simulink model "Manu6DOF_MICO_NE_v6articulation2019b"  (R2019b)
settings: Solver=ode5  StartTime=0.0  StopTime=10.0  FixedStep=0.001  RelTol=1e-3
undefined symbols (not defined in the file): f, Sub02MIHM
libraries: instrumentlib x27, dspnetwork x24, simulink x7, dspmtrx3 x3, dspsrcs4 x1
(part 3 of 3)

== matlab function Manu6DOF_MICO_NE_v6articulation2019b/Nmm to Nm ==
  data: qm input; T output
function T = fcn(qm)
%Newton milimeter to Newton meter

t1 = qm(1);
t2 = qm(2);
t3 = qm(3);
t4 = qm(4);
t5 = qm(5);
t6 = qm(6);


T = [t1*0.001;t2*0.001;t3*0.001;t4*0.001;t5*0.001;t6*0.001];

%%

== matlab function Manu6DOF_MICO_NE_v6articulation2019b/D ==
  data: qm input; M output
function M = fcn(qm)

q1 = qm(1);
q2 = qm(2);
q3 = qm(3);
q4 = qm(4);
q5 = qm(5);
q6 = qm(6);

%%%%%%%
%function M = M(q1,q2,q3,q4,q5,q6)
%D_Q

%    This function was generated by the Symbolic Math Toolbox version 8.4.
%    09-Jul-2020 20:13:24

M = reshape([conj(q1).*(-1.571066306042153e+4)-conj(q2).*4.088711718154727e+4+conj(q3).*6.059193811420593e+5+conj(q4).*2.254880071272725e+5-conj(q5).*2.343560231418765e+5+conj(q6).*2.101846903564805e+5+conj(q1).*conj(q2).*2.99983383266e+3+conj(q1).*conj(q3).*1.317626777332713e-13+conj(q1).*conj(q4).*5.296107547592644e-14+conj(q2).*conj(q3).*1.317626777332713e-13-conj(q1).*conj(q5).*4.873849331246636e-14+conj(q2).*conj(q4).*5.296107547592644e-14+conj(q1).*conj(q6).*1.335477334470189e-13-conj(q2).*conj(q5).*4.873849331246636e-14+conj(q3).*conj(q4).*8.6492e+2+conj(q2).*conj(q6).*1.335477334470189e-13-conj(q3).*conj(q5).*7.9596e+2+conj(q3).*conj(q6).*7.27e+2+conj(q4).*conj(q5).*7.9596e+2-conj(q4).*conj(q6).*7.27e+2-conj(q5).*conj(q6).*1.454e+3+conj(q1).^2.*1.68190091725e+3+conj(q2).^2.*1.49991691633e+3+conj(q3).^2.*1.07592391394e+3+conj(q4).^2.*8.6492e+2+conj(q5).^2.*7.9596e+2+conj(q6).^2.*7.27e+2+sqrt(3.0).*1.67928161329898e+7+sqrt(3.0).*conj(q1).*1.015019680000001e+4+sqrt(3.0).*conj(q2).*1.015019680000001e+4+sqrt(3.0).*conj(q3).*6.09614312e+4+sqrt(3.0).*conj(q4).*6.036768560000001e+4+sqrt(3.0).*conj(q5).*1.309327791027026e-11-sqrt(3.0).*conj(q6).*3.645574198348217e-11+sqrt(3.0).*conj(q4).^2.*2.902843497617834e-31-sqrt(3.0).*conj(q5).^2.*2.671400025856601e-31-sqrt(3.0).*conj(q6).^2.*7.319869662286102e-31-sqrt(3.0).*conj(q1).*conj(q4).*8.6492e+2-sqrt(3.0).*conj(q1).*conj(q5).*7.9596e+2-sqrt(3.0).*conj(q2).*conj(q4).*8.6492e+2+sqrt(3.0).*conj(q1).*conj(q6).*7.27e+2-sqrt(3.0).*conj(q2).*conj(q5).*7.9596e+2+sqrt(3.0).*conj(q3).*conj(q4).*5.805686995235668e-31+sqrt(3.0).*conj(q2).*conj(q6).*7.27e+2+sqrt(3.0).*conj(q3).*conj(q5).*5.342800051713201e-31-sqrt(3.0).*conj(q3).*conj(q6).*8.903182229801258e-14-sqrt(3.0).*conj(q4).*conj(q6).*8.903182229801258e-14+sqrt(3.0).*conj(q5).*conj(q6).*9.75982621638147e-31+1.141163110828982e+8,conj(q1).*(-2.044355859077363e+4)-conj(q2).*4.088711718154727e+4+conj(q3).*3.095751114833673e+5+conj(q4).*1.063745259636362e+5-conj(q5).*1.247394499709383e+5+conj(q6).*1.100650251782402e+5+conj(q1).*conj(q2).*1.49991691633e+3+conj(q1).*conj(q3).*6.588133886663567e-14+conj(q1).*conj(q4).*2.648053773796322e-14+conj(q2).*conj(q3).*1.317626777332713e-13-conj(q1).*conj(q5).*2.436924665623318e-14+conj(q2).*conj(q4).*5.296107547592644e-14+conj(q1).*conj(q6).*6.677386672350943e-14-conj(q2).*conj(q5).*4.873849331246636e-14+conj(q3).*conj(q4).*8.6492e+2+conj(q2).*conj(q6).*1.335477334470189e-13-conj(q3).*conj(q5).*7.9596e+2+conj(q3).*conj(q6).*7.27e+2+conj(q4).*conj(q5).*7.9596e+2-conj(q4).*conj(q6).*7.27e+2-conj(q5).*conj(q6).*1.454e+3+conj(q2).^2.*1.49991691633e+3+conj(q3).^2.*1.07592391394e+3+conj(q4).^2.*8.6492e+2+conj(q5).^2.*7.9596e+2+conj(q6).^2.*7.27e+2+sqrt(3.0).*8.397440506400625e+6+sqrt(3.0).*conj(q1).*5.075098400000006e+3+sqrt(3.0).*conj(q2).*1.015019680000001e+4+sqrt(3.0).*conj(q3).*6.09614312e+4+sqrt(3.0).*conj(q4).*6.036768560000001e+4+sqrt(3.0).*conj(q5).*6.381198636905707e-12-sqrt(3.0).*conj(q6).*1.806405785964667e-11+sqrt(3.0).*conj(q4).^2.*2.902843497617834e-31-sqrt(3.0).*conj(q5).^2.*2.671400025856601e-31-sqrt(3.0).*conj(q6).^2.*7.319869662286102e-31-sqrt(3.0).*conj(q1).*conj(q4).*4.3246e+2-sqrt(3.0).*conj(q1).*conj(q5).*3.9798e+2-sqrt(3.0).*conj(q2).*conj(q4).*8.6492e+2+sqrt(3.0).*conj(q1).*conj(q6).*3.635e+2-sqrt(3.0).*conj(q2).*conj(q5).*7.9596e+2+sqrt(3.0).*conj(q3).*conj(q4).*5.805686995235668e-31+sqrt(3.0).*conj(q2).*conj(q6).*7.27e+2+sqrt(3.0).*conj(q3).*conj(q5).*5.342800051713201e-31-sqrt(3.0).*conj(q3).*conj(q6).*8.903182229801258e-14-sqrt(3.0).*conj(q4).*conj(q6).*8.903182229801258e-14+sqrt(3.0).*conj(q5).*conj(q6).*9.75982621638147e-31+2.944694702731556e+7,conj(q1).*(-2.990189516772894e+4)-conj(q2).*2.990189516772894e+4+conj(q3).*3.095751114833673e+5+conj(q4).*1.063745259636362e+5-conj(q5).*1.247394499709383e+5+conj(q6).*1.100650251782402e+5+conj(q1).*conj(q3).*6.588133886663567e-14+conj(q1).*conj(q4).*2.648053773796322e-14+conj(q2).*conj(q3).*6.588133886663567e-14-conj(q1).*conj(q5).*2.436924665623318e-14+conj(q2).*conj(q4).*2.648053773796322e-14+conj(q1).*conj(q6).*6.677386672350943e-14-conj(q2).*conj(q5).*2.436924665623318e-14+conj(q3).*conj(q4).*8.6492e+2+conj(q2).*conj(q6).*6.677386672350943e-14-conj(q3).*conj(q5).*7.9596e+2+conj(q3).*conj(q6).*7.27e+2+conj(q4).*conj(q5).*7.9596e+2-conj(q4).*conj(q6).*7.27e+2-conj(q5).*conj(q6).*1.454e+3+conj(q3).^2.*1.07592391394e+3+conj(q4).^2.*8.6492e+2+conj(q5).^2.*7.9596e+2+conj(q6).^2.*7.27e+2+sqrt(3.0).*8.395359070654554e+6+sqrt(3.0).*conj(q1).*5.075098400000006e+3+sqrt(3.0).*conj(q2).*5.075098400000006e+3+sqrt(3.0).*conj(q3).*6.09614312e+4+sqrt(3.0).*conj(q4).*6.036768560000001e+4+sqrt(3.0).*conj(q5).*6.381198636905707e-12-sqrt(3.0).*conj(q6).*1.806405785964667e-11+sqrt(3.0).*conj(q4).^2.*2.902843497617834e-31-sqrt(3.0).*conj(q5).^2.*2.671400025856601e-31-sqrt(3.0).*conj(q6).^2.*7.319869662286102e-31-sqrt(3.0).*conj(q1).*conj(q4).*4.3246e+2-sqrt(3.0).*conj(q1).*conj(q5).*3.9798e+2-sqrt(3.0).*conj(q2).*conj(q4).*4.3246e+2+sqrt(3.0).*conj(q1).*conj(q6).*3.635e+2-sqrt(3.0).*conj(q2).*conj(q5).*3.9798e+2+sqrt(3.0).*conj(q3).*conj(q4).*5.805686995235668e-31+sqrt(3.0).*conj(q2).*conj(q6).*3.635e+2+sqrt(3.0).*conj(q3).*conj(q5).*5.342800051713201e-31-sqrt(3.0).*conj(q3).*conj(q6).*8.903182229801258e-14-sqrt(3.0).*conj(q4).*conj(q6).*8.903182229801258e-14+sqrt(3.0).*conj(q5).*conj(q6).*9.75982621638147e-31+7.050641110794516e+6,conj(q1).*(-2.988697e+4)-conj(q2).*2.988697e+4+conj(q3).*2.486340000000004e+3+conj(q4).*1.063745259636362e+5-conj(q5).*1.247394499709383e+5+conj(q6).*1.100650251782402e+5+conj(q1).*conj(q4).*2.648053773796322e-14-conj(q1).*conj(q5).*2.436924665623318e-14+conj(q2).*conj(q4).*2.648053773796322e-14+conj(q1).*conj(q6).*6.677386672350943e-14-conj(q2).*conj(q5).*2.436924665623318e-14+conj(q3).*conj(q4).*4.3246e+2+conj(q2).*conj(q6).*6.677386672350943e-14-conj(q3).*conj(q5).*3.9798e+2+conj(q3).*conj(q6).*3.635e+2+conj(q4).*conj(q5).*7.9596e+2-conj(q4).*conj(q6).*7.27e+2-conj(q5).*conj(q6).*1.454e+3+conj(q4).^2.*8.6492e+2+conj(q5).^2.*7.9596e+2+conj(q6).^2.*7.27e+2+sqrt(3.0).*8.395359070654554e+6+sqrt(3.0).*conj(q1).*5.075098400000006e+3+sqrt(3.0).*conj(q2).*5.075098400000006e+3+sqrt(3.0).*conj(q3).*3.04807156e+4+sqrt(3.0).*conj(q4).*6.036768560000001e+4+sqrt(3.0).*conj(q5).*6.381198636905707e-12-sqrt(3.0).*conj(q6).*1.806405785964667e-11+sqrt(3.0).*conj(q4).^2.*2.902843497617834e-31-sqrt(3.0).*conj(q5).^2.*2.671400025856601e-31-sqrt(3.0).*conj(q6).^2.*7.319869662286102e-31-sqrt(3.0).*conj(q1).*conj(q4).*4.3246e+2-sqrt(3.0).*conj(q1).*conj(q5).*3.9798e+2-sqrt(3.0).*conj(q2).*conj(q4).*4.3246e+2+sqrt(3.0).*conj(q1).*conj(q6).*3.635e+2-sqrt(3.0).*conj(q2).*conj(q5).*3.9798e+2+sqrt(3.0).*conj(q3).*conj(q4).*2.902843497617834e-31+sqrt(3.0).*conj(q2).*conj(q6).*3.635e+2+sqrt(3.0).*conj(q3).*conj(q5).*2.671400025856601e-31-sqrt(3.0).*conj(q3).*conj(q6).*4.451591114900629e-14-sqrt(3.0).*conj(q4).*conj(q6).*8.903182229801258e-14+sqrt(3.0).*conj(q5).*conj(q6).*9.75982621638147e-31+5.835208225207267e+6,conj(q1).*(-3.01838428e+4)-conj(q2).*3.01838428e+4+conj(q3).*3.780719200000004e+3-conj(q4).*3.780719200000004e+3-conj(q5).*1.247394499709383e+5+conj(q6).*1.100650251782402e+5-conj(q1).*conj(q5).*2.436924665623318e-14+conj(q1).*conj(q6).*6.677386672350943e-14-conj(q2).*conj(q5).*2.436924665623318e-14+conj(q2).*conj(q6).*6.677386672350943e-14-conj(q3).*conj(q5).*3.9798e+2+conj(q3).*conj(q6).*3.635e+2+conj(q4).*conj(q5).*3.9798e+2-conj(q4).*conj(q6).*3.635e+2-conj(q5).*conj(q6).*1.454e+3+conj(q5).^2.*7.9596e+2+conj(q6).^2.*7.27e+2+sqrt(3.0).*8.31359086279569e+6+sqrt(3.0).*conj(q1).*3.780719200000006e+3+sqrt(3.0).*conj(q2).*3.780719200000006e+3+sqrt(3.0).*conj(q3).*3.01838428e+4+sqrt(3.0).*conj(q4).*3.01838428e+4+sqrt(3.0).*conj(q5).*6.381198636905707e-12-sqrt(3.0).*conj(q6).*1.806405785964667e-11-sqrt(3.0).*conj(q5).^2.*2.671400025856601e-31-sqrt(3.0).*conj(q6).^2.*7.319869662286102e-31-sqrt(3.0).*conj(q1).*conj(q5).*3.9798e+2+sqrt(3.0).*conj(q1).*conj(q6).*3.635e+2-sqrt(3.0).*conj(q2).*conj(q5).*3.9798e+2+sqrt(3.0).*conj(q2).*conj(q6).*3.635e+2+sqrt(3.0).*conj(q3).*conj(q5).*2.671400025856601e-31-sqrt(3.0).*conj(q3).*conj(q6).*4.451591114900629e-14-sqrt(3.0).*conj(q4).*conj(q6).*4.451591114900629e-14+sqrt(3.0).*conj(q5).*conj(q6).*9.75982621638147e-31+6.090232536153054e+6,conj(q1).*(-2.988697e+4)-conj(q2).*2.988697e+4+conj(q3).*2.486340000000004e+3-conj(q4).*2.486340000000004e+3-conj(q5).*4.972680000000007e+3+conj(q6).*1.100650251782402e+5+conj(q1).*conj(q6).*6.677386672350943e-14+conj(q2).*conj(q6).*6.677386672350943e-14+conj(q3).*conj(q6).*3.635e+2-conj(q4).*conj(q6).*3.635e+2-conj(q5).*conj(q6).*7.27e+2+conj(q6).^2.*7.27e+2+sqrt(3.0).*8.231822654936826e+6+sqrt(3.0).*conj(q1).*2.486340000000006e+3+sqrt(3.0).*conj(q2).*2.486340000000006e+3+sqrt(3.0).*conj(q3).*2.988697e+4+sqrt(3.0).*conj(q4).*2.988697e+4-sqrt(3.0).*conj(q5).*1.638131320944095e-13-sqrt(3.0).*conj(q6).*1.806405785964667e-11-sqrt(3.0).*conj(q6).^2.*7.319869662286102e-31+sqrt(3.0).*conj(q1).*conj(q6).*3.635e+2+sqrt(3.0).*conj(q2).*conj(q6).*3.635e+2-sqrt(3.0).*conj(q3).*conj(q6).*4.451591114900629e-14-sqrt(3.0).*conj(q4).*conj(q6).*4.451591114900629e-14+sqrt(3.0).*conj(q5).*conj(q6).*4.879913108190735e-31+5.632229344921152e+6,conj(q1).*(-2.044355859077363e+4)-conj(q2).*4.088711718154727e+4+conj(q3).*3.095751114833673e+5+conj(q4).*1.063745259636362e+5-conj(q5).*1.247394499709383e+5+conj(q6).*1.100650251782402e+5+conj(q1).*conj(q2).*1.49991691633e+3+conj(q1).*conj(q3).*6.588133886663567e-14+conj(q1).*conj(q4).*2.648053773796322e-14+conj(q2).*conj(q3).*1.317626777332713e-13-conj(q1).*conj(q5).*2.436924665623318e-14+conj(q2).*conj(q4).*5.296107547592644e-14+conj(q1).*conj(q6).*6.677386672350943e-14-conj(q2).*conj(q5).*4.873849331246636e-14+conj(q3).*conj(q4).*8.6492e+2+conj(q2).*conj(q6).*1.335477334470189e-13-conj(q3).*conj(q5).*7.9596e+2+conj(q3).*conj(q6).*7.27e+2+conj(q4).*conj(q5).*7.9596e+2-conj(q4).*conj(q6).*7.27e+2-conj(q5).*conj(q6).*1.454e+3+conj(q2).^2.*1.49991691633e+3+conj(q3).^2.*1.07592391394e+3+conj(q4).^2.*8.6492e+2+conj(q5).^2.*7.9596e+2+conj(q6).^2.*7.27e+2+sqrt(3.0).*8.397440506400625e+6+sqrt(3.0).*conj(q1).*5.075098400000006e+3+sqrt(3.0).*conj(q2).*1.015019680000001e+4+sqrt(3.0).*conj(q3).*6.09614312e+4+sqrt(3.0).*conj(q4).*6.036768560000001e+4+sqrt(3.0).*conj(q5).*6.381198636905707e-12-sqrt(3.0).*conj(q6).*1.806405785964667e-11+sqrt(3.0).*conj(q4).^2.*2.902843497617834e-31-sqrt(3.0).*conj(q5).^2.*2.671400025856601e-31-sqrt(3.0).*conj(q6).^2.*7.319869662286102e-31-sqrt(3.0).*conj(q1).*conj(q4).*4.3246e+2-sqrt(3.0).*conj(q1).*conj(q5).*3.9798e+2-sqrt(3.0).*conj(q2).*conj(q4).*8.6492e+2+sqrt(3.0).*conj(q1).*conj(q6).*3.635e+2-sqrt(3.0).*conj(q2).*conj(q5).*7.9596e+2+sqrt(3.0).*conj(q3).*conj(q4).*5.805686995235668e-31+sqrt(3.0).*conj(q2).*conj(q6).*7.27e+2+sqrt(3.0).*conj(q3).*conj(q5).*5.342800051713201e-31-sqrt(3.0).*conj(q3).*conj(q6).*8.903182229801258e-14-sqrt(3.0).*conj(q4).*conj(q6).*8.903182229801258e-14+sqrt(3.0).*conj(q5).*conj(q6).*9.75982621638147e-31+2.944694702731556e+7,conj(q2).*(-4.088711718154727e+4)+conj(q3).*1.323084182467521e+4-conj(q4).*1.273895520000001e+4-conj(q5).*1.512287680000001e+4+conj(q6).*9.94536e+3+conj(q2).*conj(q3).*1.317626777332713e-13+conj(q2).*conj(q4).*5.296107547592644e-14-conj(q2).*conj(q5).*4.873849331246636e-14+conj(q3).*conj(q4).*8.6492e+2+conj(q2).*conj(q6).*1.335477334470189e-13-conj(q3).*conj(q5).*7.9596e+2+conj(q3).*conj(q6).*7.27e+2+conj(q4).*conj(q5).*7.9596e+2-conj(q4).*conj(q6).*7.27e+2-conj(q5).*conj(q6).*1.454e+3+conj(q2).^2.*1.49991691633e+3+conj(q3).^2.*1.07592391394e+3+conj(q4).^2.*8.6492e+2+conj(q5).^2.*7.9596e+2+conj(q6).^2.*7.27e+2+sqrt(3.0).*2.064879811453263e+3+sqrt(3.0).*conj(q2).*1.015019680000001e+4+sqrt(3.0).*conj(q3).*6.09614312e+4+sqrt(3.0).*conj(q4).*6.03676856e+4-sqrt(3.0).*conj(q5).*3.308806364588508e-13+sqrt(3.0).*conj(q6).*3.276262641888189e-13+sqrt(3.0).*conj(q4).^2.*2.902843497617834e-31-sqrt(3.0).*conj(q5).^2.*2.671400025856601e-31-sqrt(3.0).*conj(q6).^2.*7.319869662286102e-31-sqrt(3.0).*conj(q2).*conj(q4).*8.6492e+2-sqrt(3.0).*conj(q2).*conj(q5).*7.9596e+2+sqrt(3.0).*conj(q3).*conj(q4).*5.805686995235668e-31+sqrt(3.0).*conj(q2).*conj(q6).*7.27e+2+sqrt(3.0).*conj(q3).*conj(q5).*5.342800051713201e-31-sqrt(3.0).*conj(q3).*conj(q6).*8.903182229801258e-14-sqrt(3.0).*conj(q4).*conj(q6).*8.903182229801258e-14+sqrt(3.0).*conj(q5).*conj(q6).*9.75982621638147e-31+2.762484599084687e+7,conj(q2).*(-2.990189516772894e+4)+conj(q3).*1.323084182467521e+4-conj(q4).*1.273895520000001e+4-conj(q5).*1.512287680000001e+4+conj(q6).*9.94536e+3+conj(q2).*conj(q3).*6.588133886663567e-14+conj(q2).*conj(q4).*2.648053773796322e-14-conj(q2).*conj(q5).*2.436924665623318e-14+conj(q3).*conj(q4).*8.6492e+2+conj(q2).*conj(q6).*6.677386672350943e-14-conj(q3).*conj(q5).*7.9596e+2+conj(q3).*conj(q6).*7.27e+2+conj(q4).*conj(q5).*7.9596e+2-conj(q4).*conj(q6).*7.27e+2-conj(q5).*conj(q6).*1.454e+3+conj(q3).^2.*1.07592391394e+3+conj(q4).^2.*8.6492e+2+conj(q5).^2.*7.9596e+2+conj(q6).^2.*7.27e+2-sqrt(3.0).*1.655593461782811e+1+sqrt(3.0).*conj(q2).*5.075098400000006e+3+sqrt(3.0).*conj(q3).*6.09614312e+4+sqrt(3.0).*conj(q4).*6.03676856e+4-sqrt(3.0).*conj(q5).*3.308806364588508e-13+sqrt(3.0).*conj(q6).*3.276262641888189e-13+sqrt(3.0).*conj(q4).^2.*2.902843497617834e-31-sqrt(3.0).*conj(q5).^2.*2.671400025856601e-31-sqrt(3.0).*conj(q6).^2.*7.319869662286102e-31-sqrt(3.0).*conj(q2).*conj(q4).*4.3246e+2-sqrt(3.0).*conj(q2).*conj(q5).*3.9798e+2+sqrt(3.0).*conj(q3).*conj(q4).*5.805686995235668e-31+sqrt(3.0).*conj(q2).*conj(q6).*3.635e+2+sqrt(3.0).*conj(q3).*conj(q5).*5.342800051713201e-31-sqrt(3.0).*conj(q3).*conj(q6).*8.903182229801258e-14-sqrt(3.0).*conj(q4).*conj(q6).*8.903182229801258e-14+sqrt(3.0).*conj(q5).*conj(q6).*9.75982621638147e-31+5.228540074325824e+6,conj(q2).*(-2.988697e+4)+conj(q3).*2.486340000000004e+3-conj(q4).*1.273895520000001e+4-conj(q5).*1.512287680000001e+4+conj(q6).*9.94536e+3+conj(q2).*conj(q4).*2.648053773796322e-14-conj(q2).*conj(q5).*2.436924665623318e-14+conj(q3).*conj(q4).*4.3246e+2+conj(q2).*conj(q6).*6.677386672350943e-14-conj(q3).*conj(q5).*3.9798e+2+conj(q3).*conj(q6).*3.635e+2+conj(q4).*conj(q5).*7.9596e+2-conj(q4).*conj(q6).*7.27e+2-conj(q5).*conj(q6).*1.454e+3+conj(q4).^2.*8.6492e+2+conj(q5).^2.*7.9596e+2+conj(q6).^2.*7.27e+2-sqrt(3.0).*1.655593461782811e+1+sqrt(3.0).*conj(q2).*5.075098400000006e+3+sqrt(3.0).*conj(q3).*3.04807156e+4+sqrt(3.0).*conj(q4).*6.03676856e+4-sqrt(3.0).*conj(q5).*3.308806364588508e-13+sqrt(3.0).*conj(q6).*3.276262641888189e-13+sqrt(3.0).*conj(q4).^2.*2.902843497617834e-31-sqrt(3.0).*conj(q5).^2.*2.671400025856601e-31-sqrt(3.0).*conj(q6).^2.*7.319869662286102e-31-sqrt(3.0).*conj(q2).*conj(q4).*4.3246e+2-sqrt(3.0).*conj(q2).*conj(q5).*3.9798e+2+sqrt(3.0).*conj(q3).*conj(q4).*2.902843497617834e-31+sqrt(3.0).*conj(q2).*conj(q6).*3.635e+2+sqrt(3.0).*conj(q3).*conj(q5).*2.671400025856601e-31-sqrt(3.0).*conj(q3).*conj(q6).*4.451591114900629e-14-sqrt(3.0).*conj(q4).*conj(q6).*8.903182229801258e-14+sqrt(3.0).*conj(q5).*conj(q6).*9.75982621638147e-31+5.150389715388103e+6,conj(q2).*(-3.01838428e+4)+conj(q3).*3.780719200000004e+3-conj(q4).*3.780719200000004e+3-conj(q5).*1.512287680000001e+4+conj(q6).*9.94536e+3-conj(q2).*conj(q5).*2.436924665623318e-14+conj(q2).*conj(q6).*6.677386672350943e-14-conj(q3).*conj(q5).*3.9798e+2+conj(q3).*conj(q6).*3.635e+2+conj(q4).*conj(q5).*3.9798e+2-conj(q4).*conj(q6).*3.635e+2-conj(q5).*conj(q6).*1.454e+3+conj(q5).^2.*7.9596e+2+conj(q6).^2.*7.27e+2-sqrt(3.0).*1.638597635182369e+1+sqrt(3.0).*conj(q2).*3.780719200000006e+3+sqrt(3.0).*conj(q3).*3.01838428e+4+sqrt(3.0).*conj(q4).*3.01838428e+4-sqrt(3.0).*conj(q5).*3.308806364588508e-13+sqrt(3.0).*conj(q6).*3.276262641888189e-13-sqrt(3.0).*conj(q5).^2.*2.671400025856601e-31-sqrt(3.0).*conj(q6).^2.*7.319869662286102e-31-sqrt(3.0).*conj(q2).*conj(q5).*3.9798e+2+sqrt(3.0).*conj(q2).*conj(q6).*3.635e+2+sqrt(3.0).*conj(q3).*conj(q5).*2.671400025856601e-31-sqrt(3.0).*conj(q3).*conj(q6).*4.451591114900629e-14-sqrt(3.0).*conj(q4).*conj(q6).*4.451591114900629e-14+sqrt(3.0).*conj(q5).*conj(q6).*9.75982621638147e-31+5.048900100288006e+6,conj(q2).*(-2.988697e+4)+conj(q3).*2.486340000000004e+3-conj(q4).*2.486340000000004e+3-conj(q5).*4.972680000000007e+3+conj(q6).*9.94536e+3+conj(q2).*conj(q6).*6.677386672350943e-14+conj(q3).*conj(q6).*3.635e+2-conj(q4).*conj(q6).*3.635e+2-conj(q5).*conj(q6).*7.27e+2+conj(q6).^2.*7.27e+2-sqrt(3.0).*1.621601808581952e+1+sqrt(3.0).*conj(q2).*2.486340000000006e+3+sqrt(3.0).*conj(q3).*2.988697e+4+sqrt(3.0).*conj(q4).*2.988697e+4-sqrt(3.0).*conj(q5).*1.638131320944095e-13+sqrt(3.0).*conj(q6).*3.276262641888189e-13-sqrt(3.0).*conj(q6).^2.*7.319869662286102e-31+sqrt(3.0).*conj(q2).*conj(q6).*3.635e+2-sqrt(3.0).*conj(q3).*conj(q6).*4.451591114900629e-14-sqrt(3.0).*conj(q4).*conj(q6).*4.451591114900629e-14+sqrt(3.0).*conj(q5).*conj(q6).*4.879913108190735e-31+4.947410835101987e+6,conj(q1).*(-2.990189516772894e+4)-conj(q2).*2.990189516772894e+4+conj(q3).*3.095751114833673e+5+conj(q4).*1.063745259636362e+5-conj(q5).*1.247394499709383e+5+conj(q6).*1.100650251782402e+5+conj(q1).*conj(q3).*6.588133886663567e-14+conj(q1).*conj(q4).*2.648053773796322e-14+conj(q2).*conj(q3).*6.588133886663567e-14-conj(q1).*conj(q5).*2.436924665623318e-14+conj(q2).*conj(q4).*2.648053773796322e-14+conj(q1).*conj(q6).*6.677386672350943e-14-conj(q2).*conj(q5).*2.436924665623318e-14+conj(q3).*conj(q4).*8.6492e+2+conj(q2).*conj(q6).*6.677386672350943e-14-conj(q3).*conj(q5).*7.9596e+2+conj(q3).*conj(q6).*7.27e+2+conj(q4).*conj(q5).*7.9596e+2-conj(q4).*conj(q6).*7.27e+2-conj(q5).*conj(q6).*1.454e+3+conj(q3).^2.*1.07592391394e+3+conj(q4).^2.*8.6492e+2+conj(q5).^2.*7.9596e+2+conj(q6).^2.*7.27e+2+sqrt(3.0).*8.395359070654554e+6+sqrt(3.0).*conj(q1).*5.075098400000006e+3+sqrt(3.0).*conj(q2).*5.075098400000006e+3+sqrt(3.0).*conj(q3).*6.09614312e+4+sqrt(3.0).*conj(q4).*6.036768560000001e+4+sqrt(3.0).*conj(q5).*6.381198636905707e-12-sqrt(3.0).*conj(q6).*1.806405785964667e-11+sqrt(3.0).*conj(q4).^2.*2.902843497617834e-31-sqrt(3.0).*conj(q5).^2.*2.671400025856601e-31-sqrt(3.0).*conj(q6).^2.*7.319869662286102e-31-sqrt(3.0).*conj(q1).*conj(q4).*4.3246e+2-sqrt(3.0).*conj(q1).*conj(q5).*3.9798e+2-sqrt(3.0).*conj(q2).*conj(q4).*4.3246e+2+sqrt(3.0).*conj(q1).*conj(q6).*3.635e+2-sqrt(3.0).*conj(q2).*conj(q5).*3.9798e+2+sqrt(3.0).*conj(q3).*conj(q4).*5.805686995235668e-31+sqrt(3.0).*conj(q2).*conj(q6).*3.635e+2+sqrt(3.0).*conj(q3).*conj(q5).*5.342800051713201e-31-sqrt(3.0).*conj(q3).*conj(q6).*8.903182229801258e-14-sqrt(3.0).*conj(q4).*conj(q6).*8.903182229801258e-14+sqrt(3.0).*conj(q5).*conj(q6).*9.75982621638147e-31+7.050641110794516e+6,conj(q2).*(-2.990189516772894e+4)+conj(q3).*1.323084182467521e+4-conj(q4).*1.273895520000001e+4-conj(q5).*1.512287680000001e+4+conj(q6).*9.94536e+3+conj(q2).*conj(q3).*6.588133886663567e-14+conj(q2).*conj(q4).*2.648053773796322e-14-conj(q2).*conj(q5).*2.436924665623318e-14+conj(q3).*conj(q4).*8.6492e+2+conj(q2).*conj(q6).*6.677386672350943e-14-conj(q3).*conj(q5).*7.9596e+2+conj(q3).*conj(q6).*7.27e+2+conj(q4).*conj(q5).*7.9596e+2-conj(q4).*conj(q6).*7.27e+2-conj(q5).*conj(q6).*1.454e+3+conj(q3).^2.*1.07592391394e+3+conj(q4).^2.*8.6492e+2+conj(q5).^2.*7.9596e+2+conj(q6).^2.*7.27e+2-sqrt(3.0).*1.655593461782811e+1+sqrt(3.0).*conj(q2).*5.075098400000006e+3+sqrt(3.0).*conj(q3).*6.09614312e+4+sqrt(3.0).*conj(q4).*6.03676856e+4-sqrt(3.0).*conj(q5).*3.308806364588508e-13+sqrt(3.0).*conj(q6).*3.276262641888189e-13+sqrt(3.0).*conj(q4).^2.*2.902843497617834e-31-sqrt(3.0).*conj(q5).^2.*2.671400025856601e-31-sqrt(3.0).*conj(q6).^2.*7.319869662286102e-31-sqrt(3.0).*conj(q2).*conj(q4).*4.3246e+2-sqrt(3.0).*conj(q2).*conj(q5).*3.9798e+2+sqrt(3.0).*conj(q3).*conj(q4).*5.805686995235668e-31+sqrt(3.0).*conj(q2).*conj(q6).*3.635e+2+sqrt(3.0).*conj(q3).*conj(q5).*5.342800051713201e-31-sqrt(3.0).*conj(q3).*conj(q6).*8.903182229801258e-14-sqrt(3.0).*conj(q4).*conj(q6).*8.903182229801258e-14+sqrt(3.0).*conj(q5).*conj(q6).*9.75982621638147e-31+5.228540074325824e+6,conj(q3).*1.323084182467521e+4-conj(q4).*1.273895520000001e+4-conj(q5).*1.512287680000001e+4+conj(q6).*9.94536e+3+conj(q3).*conj(q4).*8.6492e+2-conj(q3).*conj(q5).*7.9596e+2+conj(q3).*conj(q6).*7.27e+2+conj(q4).*conj(q5).*7.9596e+2-conj(q4).*conj(q6).*7.27e+2-conj(q5).*conj(q6).*1.454e+3+conj(q3).^2.*1.07592391394e+3+conj(q4).^2.*8.6492e+2+conj(q5).^2.*7.9596e+2+conj(q6).^2.*7.27e+2+sqrt(3.0).*2.240963647051526e-12+sqrt(3.0).*conj(q3).*6.09614312e+4+sqrt(3.0).*conj(q4).*6.03676856e+4-sqrt(3.0).*conj(q5).*3.308806364588508e-13+sqrt(3.0).*conj(q6).*3.276262641888189e-13+sqrt(3.0).*conj(q4).^2.*2.902843497617834e-31-sqrt(3.0).*conj(q5).^2.*2.671400025856601e-31-sqrt(3.0).*conj(q6).^2.*7.319869662286102e-31+sqrt(3.0).*conj(q3).*conj(q4).*5.805686995235668e-31+sqrt(3.0).*conj(q3).*conj(q5).*5.342800051713201e-31-sqrt(3.0).*conj(q3).*conj(q6).*8.903182229801258e-14-sqrt(3.0).*conj(q4).*conj(q6).*8.903182229801258e-14+sqrt(3.0).*conj(q5).*conj(q6).*9.75982621638147e-31+5.407234478347215e+6,conj(q3).*2.486340000000004e+3-conj(q4).*1.273895520000001e+4-conj(q5).*1.512287680000001e+4+conj(q6).*9.94536e+3+conj(q3).*conj(q4).*4.3246e+2-conj(q3).*conj(q5).*3.9798e+2+conj(q3).*conj(q6).*3.635e+2+conj(q4).*conj(q5).*7.9596e+2-conj(q4).*conj(q6).*7.27e+2-conj(q5).*conj(q6).*1.454e+3+conj(q4).^2.*8.6492e+2+conj(q5).^2.*7.9596e+2+conj(q6).^2.*7.27e+2+sqrt(3.0).*2.240963647051526e-12+sqrt(3.0).*conj(q3).*3.04807156e+4+sqrt(3.0).*conj(q4).*6.03676856e+4-sqrt(3.0).*conj(q5).*3.308806364588508e-13+sqrt(3.0).*conj(q6).*3.276262641888189e-13+sqrt(3.0).*conj(q4).^2.*2.902843497617834e-31-sqrt(3.0).*conj(q5).^2.*2.671400025856601e-31-sqrt(3.0).*conj(q6).^2.*7.319869662286102e-31+sqrt(3.0).*conj(q3).*conj(q4).*2.902843497617834e-31+sqrt(3.0).*conj(q3).*conj(q5).*2.671400025856601e-31-sqrt(3.0).*conj(q3).*conj(q6).*4.451591114900629e-14-sqrt(3.0).*conj(q4).*conj(q6).*8.903182229801258e-14+sqrt(3.0).*conj(q5).*conj(q6).*9.75982621638147e-31+5.278331147904e+6,conj(q3).*3.780719200000004e+3-conj(q4).*3.780719200000004e+3-conj(q5).*1.512287680000001e+4+conj(q6).*9.94536e+3-conj(q3).*conj(q5).*3.9798e+2+conj(q3).*conj(q6).*3.635e+2+conj(q4).*conj(q5).*3.9798e+2-conj(q4).*conj(q6).*3.635e+2-conj(q5).*conj(q6).*1.454e+3+conj(q5).^2.*7.9596e+2+conj(q6).^2.*7.27e+2+sqrt(3.0).*2.363132782068523e-12+sqrt(3.0).*conj(q3).*3.01838428e+4+sqrt(3.0).*conj(q4).*3.01838428e+4-sqrt(3.0).*conj(q5).*3.308806364588508e-13+sqrt(3.0).*conj(q6).*3.276262641888189e-13-sqrt(3.0).*conj(q5).^2.*2.671400025856601e-31-sqrt(3.0).*conj(q6).^2.*7.319869662286102e-31+sqrt(3.0).*conj(q3).*conj(q5).*2.671400025856601e-31-sqrt(3.0).*conj(q3).*conj(q6).*4.451591114900629e-14-sqrt(3.0).*conj(q4).*conj(q6).*4.451591114900629e-14+sqrt(3.0).*conj(q5).*conj(q6).*9.75982621638147e-31+5.139718747952e+6,conj(q3).*2.486340000000004e+3-conj(q4).*2.486340000000004e+3-conj(q5).*4.972680000000007e+3+conj(q6).*9.94536e+3+conj(q3).*conj(q6).*3.635e+2-conj(q4).*conj(q6).*3.635e+2-conj(q5).*conj(q6).*7.27e+2+conj(q6).^2.*7.27e+2+sqrt(3.0).*2.240963647051526e-12+sqrt(3.0).*conj(q3).*2.988697e+4+sqrt(3.0).*conj(q4).*2.988697e+4-sqrt(3.0).*conj(q5).*1.638131320944095e-13+sqrt(3.0).*conj(q6).*3.276262641888189e-13-sqrt(3.0).*conj(q6).^2.*7.319869662286102e-31-sqrt(3.0).*conj(q3).*conj(q6).*4.451591114900629e-14-sqrt(3.0).*conj(q4).*conj(q6).*4.451591114900629e-14+sqrt(3.0).*conj(q5).*conj(q6).*4.879913108190735e-31+5.001106348e+6,conj(q1).*(-2.988697e+4)-conj(q2).*2.988697e+4+conj(q3).*2.486340000000004e+3+conj(q4).*1.063745259636362e+5-conj(q5).*1.247394499709383e+5+conj(q6).*1.100650251782402e+5+conj(q1).*conj(q4).*2.648053773796322e-14-conj(q1).*conj(q5).*2.436924665623318e-14+conj(q2).*conj(q4).*2.648053773796322e-14+conj(q1).*conj(q6).*6.677386672350943e-14-conj(q2).*conj(q5).*2.436924665623318e-14+conj(q3).*conj(q4).*4.3246e+2+conj(q2).*conj(q6).*6.677386672350943e-14-conj(q3).*conj(q5).*3.9798e+2+conj(q3).*conj(q6).*3.635e+2+conj(q4).*conj(q5).*7.9596e+2-conj(q4).*conj(q6).*7.27e+2-conj(q5).*conj(q6).*1.454e+3+conj(q4).^2.*8.6492e+2+conj(q5).^2.*7.9596e+2+conj(q6).^2.*7.27e+2+sqrt(3.0).*8.395359070654554e+6+sqrt(3.0).*conj(q1).*5.075098400000006e+3+sqrt(3.0).*conj(q2).*5.075098400000006e+3+sqrt(3.0).*conj(q3).*3.04807156e+4+sqrt(3.0).*conj(q4).*6.036768560000001e+4+sqrt(3.0).*conj(q5).*6.381198636905707e-12-sqrt(3.0).*conj(q6).*1.806405785964667e-11+sqrt(3.0).*conj(q4).^2.*2.902843497617834e-31-sqrt(3.0).*conj(q5).^2.*2.671400025856601e-31-sqrt(3.0).*conj(q6).^2.*7.319869662286102e-31-sqrt(3.0).*conj(q1).*conj(q4).*4.3246e+2-sqrt(3.0).*conj(q1).*conj(q5).*3.9798e+2-sqrt(3.0).*conj(q2).*conj(q4).*4.3246e+2+sqrt(3.0).*conj(q1).*conj(q6).*3.635e+2-sqrt(3.0).*conj(q2).*conj(q5).*3.9798e+2+sqrt(3.0).*conj(q3).*conj(q4).*2.902843497617834e-31+sqrt(3.0).*conj(q2).*conj(q6).*3.635e+2+sqrt(3.0).*conj(q3).*conj(q5).*2.671400025856601e-31-sqrt(3.0).*conj(q3).*conj(q6).*4.451591114900629e-14-sqrt(3.0).*conj(q4).*conj(q6).*8.903182229801258e-14+sqrt(3.0).*conj(q5).*conj(q6).*9.75982621638147e-31+5.835208225207267e+6,conj(q2).*(-2.988697e+4)+conj(q3).*2.486340000000004e+3-conj(q4).*1.273895520000001e+4-conj(q5).*1.512287680000001e+4+conj(q6).*9.94536e+3+conj(q2).*conj(q4).*2.648053773796322e-14-conj(q2).*conj(q5).*2.436924665623318e-14+conj(q3).*conj(q4).*4.3246e+2+conj(q2).*conj(q6).*6.677386672350943e-14-conj(q3).*conj(q5).*3.9798e+2+conj(q3).*conj(q6).*3.635e+2+conj(q4).*conj(q5).*7.9596e+2-conj(q4).*conj(q6).*7.27e+2-conj(q5).*conj(q6).*1.454e+3+conj(q4).^2.*8.6492e+2+conj(q5).^2.*7.9596e+2+conj(q6).^2.*7.27e+2-sqrt(3.0).*1.655593461782811e+1+sqrt(3.0).*conj(q2).*5.075098400000006e+3+sqrt(3.0).*conj(q3).*3.04807156e+4+sqrt(3.0).*conj(q4).*6.03676856e+4-sqrt(3.0).*conj(q5).*3.308806364588508e-13+sqrt(3.0).*conj(q6).*3.276262641888189e-13+sqrt(3.0).*conj(q4).^2.*2.902843497617834e-31-sqrt(3.0).*conj(q5).^2.*2.671400025856601e-31-sqrt(3.0).*conj(q6).^2.*7.319869662286102e-31-sqrt(3.0).*conj(q2).*conj(q4).*4.3246e+2-sqrt(3.0).*conj(q2).*conj(q5).*3.9798e+2+sqrt(3.0).*conj(q3).*conj(q4).*2.902843497617834e-31+sqrt(3.0).*conj(q2).*conj(q6).*3.635e+2+sqrt(3.0).*conj(q3).*conj(q5).*2.671400025856601e-31-sqrt(3.0).*conj(q3).*conj(q6).*4.451591114900629e-14-sqrt(3.0).*conj(q4).*conj(q6).*8.903182229801258e-14+sqrt(3.0).*conj(q5).*conj(q6).*9.75982621638147e-31+5.150389715388103e+6,conj(q3).*2.486340000000004e+3-conj(q4).*1.273895520000001e+4-conj(q5).*1.512287680000001e+4+conj(q6).*9.94536e+3+conj(q3).*conj(q4).*4.3246e+2-conj(q3).*conj(q5).*3.9798e+2+conj(q3).*conj(q6).*3.635e+2+conj(q4).*conj(q5).*7.9596e+2-conj(q4).*conj(q6).*7.27e+2-conj(q5).*conj(q6).*1.454e+3+conj(q4).^2.*8.6492e+2+conj(q5).^2.*7.9596e+2+conj(q6).^2.*7.27e+2+sqrt(3.0).*2.240963647051526e-12+sqrt(3.0).*conj(q3).*3.04807156e+4+sqrt(3.0).*conj(q4).*6.03676856e+4-sqrt(3.0).*conj(q5).*3.308806364588508e-13+sqrt(3.0).*conj(q6).*3.276262641888189e-13+sqrt(3.0).*conj(q4).^2.*2.902843497617834e-31-sqrt(3.0).*conj(q5).^2.*2.671400025856601e-31-sqrt(3.0).*conj(q6).^2.*7.319869662286102e-31+sqrt(3.0).*conj(q3).*conj(q4).*2.902843497617834e-31+sqrt(3.0).*conj(q3).*conj(q5).*2.671400025856601e-31-sqrt(3.0).*conj(q3).*conj(q6).*4.451591114900629e-14-sqrt(3.0).*conj(q4).*conj(q6).*8.903182229801258e-14+sqrt(3.0).*conj(q5).*conj(q6).*9.75982621638147e-31+5.278331147904e+6,conj(q4).*(-1.273895520000001e+4)-conj(q5).*1.512287680000001e+4+conj(q6).*9.94536e+3+conj(q4).*conj(q5).*7.9596e+2-conj(q4).*conj(q6).*7.27e+2-conj(q5).*conj(q6).*1.454e+3+conj(q4).^2.*8.6492e+2+conj(q5).^2.*7.9596e+2+conj(q6).^2.*7.27e+2+sqrt(3.0).*2.240963647051526e-12+sqrt(3.0).*conj(q4).*6.03676856e+4-sqrt(3.0).*conj(q5).*3.308806364588508e-13+sqrt(3.0).*conj(q6).*3.276262641888189e-13+sqrt(3.0).*conj(q4).^2.*2.902843497617834e-31-sqrt(3.0).*conj(q5).^2.*2.671400025856601e-31-sqrt(3.0).*conj(q6).^2.*7.319869662286102e-31-sqrt(3.0).*conj(q4).*conj(q6).*8.903182229801258e-14+sqrt(3.0).*conj(q5).*conj(q6).*9.75982621638147e-31+5.278331147904e+6,conj(q4).*(-3.780719200000004e+3)-conj(q5).*1.512287680000001e+4+conj(q6).*9.94536e+3+conj(q4).*conj(q5).*3.9798e+2-conj(q4).*conj(q6).*3.635e+2-conj(q5).*conj(q6).*1.454e+3+conj(q5).^2.*7.9596e+2+conj(q6).^2.*7.27e+2+sqrt(3.0).*2.363132782068523e-12+sqrt(3.0).*conj(q4).*3.01838428e+4-sqrt(3.0).*conj(q5).*3.308806364588508e-13+sqrt(3.0).*conj(q6).*3.276262641888189e-13-sqrt(3.0).*conj(q5).^2.*2.671400025856601e-31-sqrt(3.0).*conj(q6).^2.*7.319869662286102e-31-sqrt(3.0).*conj(q4).*conj(q6).*4.451591114900629e-14+sqrt(3.0).*conj(q5).*conj(q6).*9.75982621638147e-31+5.139718747952e+6,conj(q4).*(-2.486340000000004e+3)-conj(q5).*4.972680000000007e+3+conj(q6).*9.94536e+3-conj(q4).*conj(q6).*3.635e+2-conj(q5).*conj(q6).*7.27e+2+conj(q6).^2.*7.27e+2+sqrt(3.0).*2.240963647051526e-12+sqrt(3.0).*conj(q4).*2.988697e+4-sqrt(3.0).*conj(q5).*1.638131320944095e-13+sqrt(3.0).*conj(q6).*3.276262641888189e-13-sqrt(3.0).*conj(q6).^2.*7.319869662286102e-31-sqrt(3.0).*conj(q4).*conj(q6).*4.451591114900629e-14+sqrt(3.0).*conj(q5).*conj(q6).*4.879913108190735e-31+5.001106348e+6,conj(q1).*(-3.01838428e+4)-conj(q2).*3.01838428e+4+conj(q3).*3.780719200000004e+3-conj(q4).*3.780719200000004e+3-conj(q5).*1.247394499709383e+5+conj(q6).*1.100650251782402e+5-conj(q1).*conj(q5).*2.436924665623318e-14+conj(q1).*conj(q6).*6.677386672350943e-14-conj(q2).*conj(q5).*2.436924665623318e-14+conj(q2).*conj(q6).*6.677386672350943e-14-conj(q3).*conj(q5).*3.9798e+2+conj(q3).*conj(q6).*3.635e+2+conj(q4).*conj(q5).*3.9798e+2-conj(q4).*conj(q6).*3.635e+2-conj(q5).*conj(q6).*1.454e+3+conj(q5).^2.*7.9596e+2+conj(q6).^2.*7.27e+2+sqrt(3.0).*8.31359086279569e+6+sqrt(3.0).*conj(q1).*3.780719200000006e+3+sqrt(3.0).*conj(q2).*3.780719200000006e+3+sqrt(3.0).*conj(q3).*3.01838428e+4+sqrt(3.0).*conj(q4).*3.01838428e+4+sqrt(3.0).*conj(q5).*6.381198636905707e-12-sqrt(3.0).*conj(q6).*1.806405785964667e-11-sqrt(3.0).*conj(q5).^2.*2.671400025856601e-31-sqrt(3.0).*conj(q6).^2.*7.319869662286102e-31-sqrt(3.0).*conj(q1).*conj(q5).*3.9798e+2+sqrt(3.0).*conj(q1).*conj(q6).*3.635e+2-sqrt(3.0).*conj(q2).*conj(q5).*3.9798e+2+sqrt(3.0).*conj(q2).*conj(q6).*3.635e+2+sqrt(3.0).*conj(q3).*conj(q5).*2.671400025856601e-31-sqrt(3.0).*conj(q3).*conj(q6).*4.451591114900629e-14-sqrt(3.0).*conj(q4).*conj(q6).*4.451591114900629e-14+sqrt(3.0).*conj(q5).*conj(q6).*9.75982621638147e-31+6.090232536153054e+6,conj(q2).*(-3.01838428e+4)+conj(q3).*3.780719200000004e+3-conj(q4).*3.780719200000004e+3-conj(q5).*1.512287680000001e+4+conj(q6).*9.94536e+3-conj(q2).*conj(q5).*2.436924665623318e-14+conj(q2).*conj(q6).*6.677386672350943e-14-conj(q3).*conj(q5).*3.9798e+2+conj(q3).*conj(q6).*3.635e+2+conj(q4).*conj(q5).*3.9798e+2-conj(q4).*conj(q6).*3.635e+2-conj(q5).*conj(q6).*1.454e+3+conj(q5).^2.*7.9596e+2+conj(q6).^2.*7.27e+2-sqrt(3.0).*1.638597635182369e+1+sqrt(3.0).*conj(q2).*3.780719200000006e+3+sqrt(3.0).*conj(q3).*3.01838428e+4+sqrt(3.0).*conj(q4).*3.01838428e+4-sqrt(3.0).*conj(q5).*3.308806364588508e-13+sqrt(3.0).*conj(q6).*3.276262641888189e-13-sqrt(3.0).*conj(q5).^2.*2.671400025856601e-31-sqrt(3.0).*conj(q6).^2.*7.319869662286102e-31-sqrt(3.0).*conj(q2).*conj(q5).*3.9798e+2+sqrt(3.0).*conj(q2).*conj(q6).*3.635e+2+sqrt(3.0).*conj(q3).*conj(q5).*2.671400025856601e-31-sqrt(3.0).*conj(q3).*conj(q6).*4.451591114900629e-14-sqrt(3.0).*conj(q4).*conj(q6).*4.451591114900629e-14+sqrt(3.0).*conj(q5).*conj(q6).*9.75982621638147e-31+5.048900100288006e+6,conj(q3).*3.780719200000004e+3-conj(q4).*3.780719200000004e+3-conj(q5).*1.512287680000001e+4+conj(q6).*9.94536e+3-conj(q3).*conj(q5).*3.9798e+2+conj(q3).*conj(q6).*3.635e+2+conj(q4).*conj(q5).*3.9798e+2-conj(q4).*conj(q6).*3.635e+2-conj(q5).*conj(q6).*1.454e+3+conj(q5).^2.*7.9596e+2+conj(q6).^2.*7.27e+2+sqrt(3.0).*2.363132782068523e-12+sqrt(3.0).*conj(q3).*3.01838428e+4+sqrt(3.0).*conj(q4).*3.01838428e+4-sqrt(3.0).*conj(q5).*3.308806364588508e-13+sqrt(3.0).*conj(q6).*3.276262641888189e-13-sqrt(3.0).*conj(q5).^2.*2.671400025856601e-31-sqrt(3.0).*conj(q6).^2.*7.319869662286102e-31+sqrt(3.0).*conj(q3).*conj(q5).*2.671400025856601e-31-sqrt(3.0).*conj(q3).*conj(q6).*4.451591114900629e-14-sqrt(3.0).*conj(q4).*conj(q6).*4.451591114900629e-14+sqrt(3.0).*conj(q5).*conj(q6).*9.75982621638147e-31+5.139718747952e+6,conj(q4).*(-3.780719200000004e+3)-conj(q5).*1.512287680000001e+4+conj(q6).*9.94536e+3+conj(q4).*conj(q5).*3.9798e+2-conj(q4).*conj(q6).*3.635e+2-conj(q5).*conj(q6).*1.454e+3+conj(q5).^2.*7.9596e+2+conj(q6).^2.*7.27e+2+sqrt(3.0).*2.363132782068523e-12+sqrt(3.0).*conj(q4).*3.01838428e+4-sqrt(3.0).*conj(q5).*3.308806364588508e-13+sqrt(3.0).*conj(q6).*3.276262641888189e-13-sqrt(3.0).*conj(q5).^2.*2.671400025856601e-31-sqrt(3.0).*conj(q6).^2.*7.319869662286102e-31-sqrt(3.0).*conj(q4).*conj(q6).*4.451591114900629e-14+sqrt(3.0).*conj(q5).*conj(q6).*9.75982621638147e-31+5.139718747952e+6,conj(q5).*(-1.512287680000001e+4)+conj(q6).*9.94536e+3-conj(q5).*conj(q6).*1.454e+3+conj(q5).^2.*7.9596e+2+conj(q6).^2.*7.27e+2+sqrt(3.0).*2.363132782068523e-12-sqrt(3.0).*conj(q5).*3.308806364588508e-13+sqrt(3.0).*conj(q6).*3.276262641888189e-13-sqrt(3.0).*conj(q5).^2.*2.671400025856601e-31-sqrt(3.0).*conj(q6).^2.*7.319869662286102e-31+sqrt(3.0).*conj(q5).*conj(q6).*9.75982621638147e-31+5.139718747952e+6,conj(q5).*(-4.972680000000007e+3)+conj(q6).*9.94536e+3-conj(q5).*conj(q6).*7.27e+2+conj(q6).^2.*7.27e+2+sqrt(3.0).*2.240963647051526e-12-sqrt(3.0).*conj(q5).*1.638131320944095e-13+sqrt(3.0).*conj(q6).*3.276262641888189e-13-sqrt(3.0).*conj(q6).^2.*7.319869662286102e-31+sqrt(3.0).*conj(q5).*conj(q6).*4.879913108190735e-31+5.001106348e+6,conj(q1).*(-2.988697e+4)-conj(q2).*2.988697e+4+conj(q3).*2.486340000000004e+3-conj(q4).*2.486340000000004e+3-conj(q5).*4.972680000000007e+3+conj(q6).*1.100650251782402e+5+conj(q1).*conj(q6).*6.677386672350943e-14+conj(q2).*conj(q6).*6.677386672350943e-14+conj(q3).*conj(q6).*3.635e+2-conj(q4).*conj(q6).*3.635e+2-conj(q5).*conj(q6).*7.27e+2+conj(q6).^2.*7.27e+2+sqrt(3.0).*8.231822654936826e+6+sqrt(3.0).*conj(q1).*2.486340000000006e+3+sqrt(3.0).*conj(q2).*2.486340000000006e+3+sqrt(3.0).*conj(q3).*2.988697e+4+sqrt(3.0).*conj(q4).*2.988697e+4-sqrt(3.0).*conj(q5).*1.638131320944095e-13-sqrt(3.0).*conj(q6).*1.806405785964667e-11-sqrt(3.0).*conj(q6).^2.*7.319869662286102e-31+sqrt(3.0).*conj(q1).*conj(q6).*3.635e+2+sqrt(3.0).*conj(q2).*conj(q6).*3.635e+2-sqrt(3.0).*conj(q3).*conj(q6).*4.451591114900629e-14-sqrt(3.0).*conj(q4).*conj(q6).*4.451591114900629e-14+sqrt(3.0).*conj(q5).*conj(q6).*4.879913108190735e-31+5.632229344921152e+6,conj(q2).*(-2.988697e+4)+conj(q3).*2.486340000000004e+3-conj(q4).*2.486340000000004e+3-conj(q5).*4.972680000000007e+3+conj(q6).*9.94536e+3+conj(q2).*conj(q6).*6.677386672350943e-14+conj(q3).*conj(q6).*3.635e+2-conj(q4).*conj(q6).*3.635e+2-conj(q5).*conj(q6).*7.27e+2+conj(q6).^2.*7.27e+2-sqrt(3.0).*1.621601808581952e+1+sqrt(3.0).*conj(q2).*2.486340000000006e+3+sqrt(3.0).*conj(q3).*2.988697e+4+sqrt(3.0).*conj(q4).*2.988697e+4-sqrt(3.0).*conj(q5).*1.638131320944095e-13+sqrt(3.0).*conj(q6).*3.276262641888189e-13-sqrt(3.0).*conj(q6).^2.*7.319869662286102e-31+sqrt(3.0).*conj(q2).*conj(q6).*3.635e+2-sqrt(3.0).*conj(q3).*conj(q6).*4.451591114900629e-14-sqrt(3.0).*conj(q4).*conj(q6).*4.451591114900629e-14+sqrt(3.0).*conj(q5).*conj(q6).*4.879913108190735e-31+4.947410835101987e+6,conj(q3).*2.486340000000004e+3-conj(q4).*2.486340000000004e+3-conj(q5).*4.972680000000007e+3+conj(q6).*9.94536e+3+conj(q3).*conj(q6).*3.635e+2-conj(q4).*conj(q6).*3.635e+2-conj(q5).*conj(q6).*7.27e+2+conj(q6).^2.*7.27e+2+sqrt(3.0).*2.240963647051526e-12+sqrt(3.0).*conj(q3).*2.988697e+4+sqrt(3.0).*conj(q4).*2.988697e+4-sqrt(3.0).*conj(q5).*1.638131320944095e-13+sqrt(3.0).*conj(q6).*3.276262641888189e-13-sqrt(3.0).*conj(q6).^2.*7.319869662286102e-31-sqrt(3.0).*conj(q3).*conj(q6).*4.451591114900629e-14-sqrt(3.0).*conj(q4).*conj(q6).*4.451591114900629e-14+sqrt(3.0).*conj(q5).*conj(q6).*4.879913108190735e-31+5.001106348e+6,conj(q4).*(-2.486340000000004e+3)-conj(q5).*4.972680000000007e+3+conj(q6).*9.94536e+3-conj(q4).*conj(q6).*3.635e+2-conj(q5).*conj(q6).*7.27e+2+conj(q6).^2.*7.27e+2+sqrt(3.0).*2.240963647051526e-12+sqrt(3.0).*conj(q4).*2.988697e+4-sqrt(3.0).*conj(q5).*1.638131320944095e-13+sqrt(3.0).*conj(q6).*3.276262641888189e-13-sqrt(3.0).*conj(q6).^2.*7.319869662286102e-31-sqrt(3.0).*conj(q4).*conj(q6).*4.451591114900629e-14+sqrt(3.0).*conj(q5).*conj(q6).*4.879913108190735e-31+5.001106348e+6,conj(q5).*(-4.972680000000007e+3)+conj(q6).*9.94536e+3-conj(q5).*conj(q6).*7.27e+2+conj(q6).^2.*7.27e+2+sqrt(3.0).*2.240963647051526e-12-sqrt(3.0).*conj(q5).*1.638131320944095e-13+sqrt(3.0).*conj(q6).*3.276262641888189e-13-sqrt(3.0).*conj(q6).^2.*7.319869662286102e-31+sqrt(3.0).*conj(q5).*conj(q6).*4.879913108190735e-31+5.001106348e+6,conj(q6).*9.94536e+3+conj(q6).^2.*7.27e+2+sqrt(3.0).*2.240963647051526e-12+sqrt(3.0).*conj(q6).*3.276262641888189e-13-sqrt(3.0).*conj(q6).^2.*7.319869662286102e-31+5.001106348e+6],[6,6]);


%%%%%%%%%%%%%%%
%%

== matlab function Manu6DOF_MICO_NE_v6articulation2019b/g ==
  data: qm input; G output
function G = fcn(qm)

theta_1 = qm(1);
theta_2 = qm(2);
theta_3 = qm(3);
theta_4 = qm(4);
theta_5 = qm(5);
theta_6 = qm(6);

disp theta_1 theta_2  theta_3  theta_4  theta_5  theta_6 
%%%%%%%%%%%%%%%%%%%%%%%
%G_Q


%    This function was generated by the Symbolic Math Toolbox version 8.4.
%    09-Jul-2020 18:50:18

G = [0.0;0.0;1.054861899110132e+7;sqrt(3.0).*2.596216141849145e-10+4.239942722516781e+6;sqrt(3.0).*2.389220043780056e-10-3.901892440242401e+6;sqrt(3.0).*(-6.546671837132898e-10)+3.56384215796802e+6];
%%%%%%%%%%%%%%%%%%%

== matlab function Manu6DOF_MICO_NE_v6articulation2019b/NE Torque Computation ==
  data: jointTorques output; paramList input; paramListDot input; paramListDDot input
% FUNCTION NAME : newtonEuler
% DESCRIPTION   : This function computes the inverse dynamics of a serial link manipulator
%                 and provides the velocity jacobian and its rate of change.
%
% OUTPUT        : The output gives the the joint torques at each joint,
%                 velocity Jacobian and time derivative of velocity
%                 Jacobian.
%
% INPUT         : The inputs are a list of joint parameters created
%                 with createLink,the the current joint angles/distances,
%                 the current joint angle/distance speeds,
%                 the current joint angle/distance accelerations and
%                 the boundary conditions corresponding to angular
%                 velocity, angular acceleration, linear acceleration,
%                 force and torque.
%UNITS: mm deg sec Nmm
%all the information from the spreadsheet
function jointTorques  = newtonEuler( paramList, paramListDot, paramListDDot )
N=6; %Number of links
a = zeros(N,1);
d = zeros(N,1);
alpha = zeros(N,1);
theta = zeros(N,1);
% isRotary = zeros(6,1);
J_Inertia = zeros(3,3,N);
theta_dot = zeros(N,1);
theta_ddot = zeros(N,1);
d_dot = zeros(N,1);%Linear Velocity
d_ddot = zeros(N,1); %Linear acceleration
J = zeros(3,3,N); % what is this
rcom = zeros(3,N);
rcom_base = zeros(3,N);% what is this
m = zeros(N,1);% What is this
jointTorques = zeros(N,1);

%Inertias
%% Matrix of inertia for each link
% Moment of inertia taken from manufacturer (grams*mm^2)
Lxx = 102070.25511638;  Lxy = -5.21439353;      Lxz = -21186.54126343;
Lyx = -5.21439353;      Lyy = 324893.60122828;  Lyz = -4.14134763;
Lzx = -21186.54126343;  Lzy = -4.14134763;      Lzz = 353694.43212892;
li1 = ([Lxx,Lxy,Lxz;Lyx,Lyy,Lyz;Lzx,Lzy,Lzz]);

%link2
Lxx = 3786230.46078145; Lxy = 0.00000000;       Lxz = 0.00000000;
Lyx = 0.00000000;       Lyy = 3725126.44653966; Lyz = -59.03745106;
Lzx = 0.00000000;       Lzy = -59.03745106;     Lzz = 69776.66770227;
li2 = ([Lxx,Lxy,Lxz;Lyx,Lyy,Lyz;Lzx,Lzy,Lzz]);

%link3:
Lxx = 510995.83838128;  Lxy = 1.92269188;       Lxz = -1586.22384686;
Lyx = 1.92269188;       Lyy = 480446.67577576;  Lyz = 1.96023437;
Lzx = -1586.22384686;   Lzy = 1.96023437;       Lzz = 48101.36036170;
li3 = ([Lxx,Lxy,Lxz;Lyx,Lyy,Lyz;Lzx,Lzy,Lzz]);

%link4:
Lxx = 24561.75;         Lxy = 8328.79;          Lxz = 0.35;
Lyx = 8328.79;          Lyy = 34174.42;         Lyz = 0.34;
Lzx = 0.35;             Lzy = 0.34;             Lzz = 36318.26;
li4 = ([Lxx,Lxy,Lxz;Lyx,Lyy,Lyz;Lzx,Lzy,Lzz]);

%link5:
li5 =([Lxx,Lxy,Lxz;Lyx,Lyy,Lyz;Lzx,Lzy,Lzz]);

%link6: (hand)
Lxx = 46596.24;         Lxy = 4130.32;          Lxz = -105.73;
Lyx = 4130.32;          Lyy = 26473.06;         Lyz = -32.44;
Lzx = -105.73;          Lzy = -32.44;           Lzz = 52479.87;
li6 =([Lxx,Lxy,Lxz;Lyx,Lyy,Lyz;Lzx,Lzy,Lzz]);
%%%


%%%
%L = createLink(a, d, alpha, theta, centerOfMass, mass, inertia) 
linkList=repmat(createLink(0,0.2755,pi/2,[],[69.17216347;-0.23712255;-10.29160997],181.98400092,(li1)),[N,1]);  %link 1 %dh %centerof mass %inertia 
linkList(1)=createLink(0,275.5,pi/2,[],[69.17216347;-0.23712255;-10.29160997],181.98400092,(li1));             %link 1 %dh %centerof mass %inertia 
linkList(2)=createLink(410,0,0,[],[22.30776575;0.02629337;-205.23664355],423.99300239,(li2));                    %link 2 %dh %centerof mass %inertia 
linkList(3)=createLink(0,-980,pi/2,[],[19.56874086;0.07073408;-64.37250505],211.00391394,(li3));                 %link 3 %dh %centerof mass %inertia 
linkList(4)=createLink(0,-315.8,pi/3,[],[-37.54;-8.61;0.00],68.96,(li4));             %link 4 %dh %centerof mass %inertia 
linkList(5)=createLink(0,-85.6,pi/3,[],[-37.54;-8.61;0.00],68.96,(li5));                    %link 5 %dh %centerof mass %inertia 
linkList(6)=createLink(0,-202.8,pi,[],[6.84;82.22;0.03],727.00,(li6));                 %link 6 %dh %centerof mass %inertia 

boundary_conditions = struct('angV',zeros(3,1),'linA',zeros(3,1),'angA',zeros(3,1));
boundary_conditions.base_angular_velocity = [0;0;0];
boundary_conditions.base_linear_acceleration = [0;0;-9.8];
boundary_conditions.base_angular_acceleration= [0;0;0];
boundary_conditions.distal_force = [0;0;0];
boundary_conditions.distal_torque = [0;0;0];
T = zeros(4,4,N); %Transformation
dd = zeros(3,N+1); % displacement vector in the homogenous matrix
Z = zeros(3,N+1); % Direction of Z
w = zeros(3,N+1); %Angular velocities
dd_dot = zeros(3,N+1);
H = eye(4);
w_dot = zeros(3,N+1);
dd_ddot = zeros(3,N+1);
rcom_base_dot = zeros(3,N);
rcom_base_ddot = zeros(3,N);
f = zeros(3,N+1);
n = zeros(3,N+1);
R=zeros(3,3,6);

for i = 1:N
    a(i) = linkList(i).a;
    alpha(i) = linkList(i).alpha;
    d(i) = linkList(i).d;
    theta(i) = paramList(i);
    theta_dot(i) = paramListDot(i);
    theta_ddot(i) = paramListDDot(i);
    J_Inertia(:,:,i) = linkList(i).inertia;
    rcom(:,i) = linkList(i).com;
    m(i) = linkList(i).mass;
end


for i = 1:N
    T(:,:,i) = zeros(4,4);
end

dd(:,1) = [0; 0; 0];
Z(:,1) = [0; 0; 1];

for i = 1:N
    T(:,:,i)=H*dhTransform(a(i),d(i),alpha(i),theta(i));
    H = T(:,:,i);
end

for i = 2:N+1
    dd(:,i) = T(1:3,4,i-1);
    Z(:,i) = T(1:3,3,i-1);
    R(:,:,i-1) = T(1:3,1:3,i-1);
end

for i = 1:N
    J(:,:,i) = R(:,:,i)*J_Inertia(:,:,i)*R(:,:,i)';
end
%----------------------------------------------------

w(:,1) = boundary_conditions(1).base_angular_velocity;

for i = 2:N+1

        w(:,i) = w(:,i-1) + theta_dot(i-1)*Z(:,i-1);

end


w_dot(:,1) = boundary_conditions(1).base_angular_acceleration;


    w_dot(:,2) = w_dot(:,1) + theta_ddot(1)*Z(:,1) + cross(w(:,1),Z(:,1));


for i = 3:N+1

        w_dot(:,i) = w_dot(:,i-1) + theta_ddot(i-1)*Z(:,i-1) + cross(w(:,i-1),w(:,i));

end

dd_dot(:,1) = [0; 0; 0];
for i = 2:N+1

        dd_dot(:,i) = dd_dot(:,i-1) + cross(w(:,i),(dd(:,i)-dd(:,i-1)));

end


dd_ddot(:,1) = boundary_conditions(1).base_linear_acceleration;

for i = 2:N+1

        dd_ddot(:,i:i) = dd_ddot(:,i-1) + cross(w_dot(:,i),(dd(:,i)-dd(:,i-1))) + cross(w(:,i),cross(w(:,i),(dd(:,i)-dd(:,i-1))));

end



for i = 1:N
    rcom_base(:,i) = R(:,:,i)*rcom(:,i);
end



for i = 1:N

        rcom_base_dot(:,i) = dd_dot(:,i) + cross(w(:,i+1),rcom(:,i));

end





for i = 1:N

        rcom_base_ddot(:,i) = dd_ddot(:,i) + cross(w_dot(:,i+1),(dd(:,i+1)-dd(:,i)+rcom_base(:,i))) + cross(w(:,i+1),cross(w(:,i+1),(dd(:,i+1)-dd(:,i)+rcom_base(:,i))));

end
%force torque calc

f(:,N+1) = boundary_conditions(1).distal_force;
n(:,N+1) = boundary_conditions(1).distal_torque;
for i = N:-1:1
    
    f(:,i) = f(:,i+1) + m(i)*rcom_base_ddot(:,i);
    n(:,i) = n(:,i+1) + cross(dd(:,i+1)-dd(:,i)+rcom_base(:,i),f(:,i)) + J(:,:,i)*w_dot(:,i+1) + cross(w(:,i+1),J(:,:,i)*w(:,i+1)) - cross(rcom_base(:,i),f(:,i+1));
    

        jointTorques(i,1) = Z(:,i).'*n(:,i);  %Newton milimeters

end
end
